simulink model "gyro_test"  (R2015a)
settings: Solver=ode3  StartTime=0.0  StopTime=inf  RelTol=1e-3
libraries: arduinolib x1
settings Model: SimulationMode=external  ExtModeTrigDuration=2  Creator=shohei  LastModifiedBy=shohei
settings OptimizationCC: OptimizeModelRefInitCode=on  LifeSpan=1
settings DebuggingCC: UnderspecifiedInitializationDetection=Classic  MergeDetectMultiDrivingBlocksExec=none
settings HardwareCC: ProdBitPerInt=16  ProdBitPerPointer=8  ProdIntDivRoundTo=Zero  ProdEndianess=LittleEndian  ProdWordSize=8  ProdHWDeviceType=Atmel->AVR
settings RTWCC: SystemTargetFile=realtime.tlc  GenerateMakefile=off  TemplateMakefile=realtime.tmf  Description=Run on Target Hardware  RTWVerbose=off
settings ERTTargetCC: CombineOutputUpdateFcns=off  ExtModeTransport=3  ExtModeMexFile=ext_serial_win32_comm_rtt  ExtModeMexArgs=0 1 9600  ERTSrcFileBannerTemplate=realtime_code_template.cgt  ERTHdrFileBannerTemplate=realtime_code_template.cgt  ERTDataSrcFileTemplate=realtime_code_template.cgt  ERTDataHdrFileTemplate=realtime_code_template.cgt  ERTCustomFileTemplate=realtime_file_process.tlc

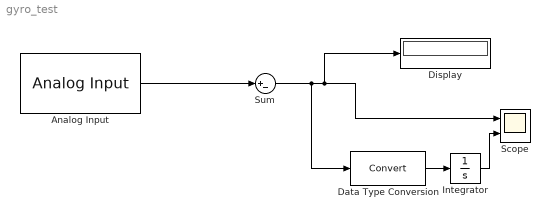
== system gyro_test ==
  Analog Input : arduinolib/Analog Input  pinNumber=5  sampleTime=0.01  blockPlatform=arduino
  Data Type Conversion : DataTypeConversion
  Display : Display
  Integrator : Integrator
  Scope : Scope  NumInputPorts=2
      settings: YMin=0~0  YMax=1023~1000
  Sum : Sum  Inputs=|+-
  wires:
  Integrator/1 -> Scope/2
  Data Type Conversion/1 -> Integrator/1
  Analog Input/1 -> Sum/1
  Sum/1 -> Data Type Conversion/1, Display/1, Scope/1
